simulink model "Saturation_Dynamic_verif"  (Simulink 7.2)
settings: Solver=ode45  StartTime=0.0  StopTime=10.0  RelTol=1e-3
libraries: simulink x1
settings Model: Creator=Romain  LastModifiedBy=Romain
settings OptimizationCC: ExpressionDepthLimit=128
settings DebuggingCC: SolverPrmCheckMsg=none  FcnCallInpInsideContextMsg=Enable All  StateNameClashWarn=none  StrictBusMsg=ErrorLevel1
settings CodeAppCC: CustomSymbolStrType=$N$R$M_T
settings GRTTargetCC: TargetFunctionLibrary=C89/C90 (ANSI)

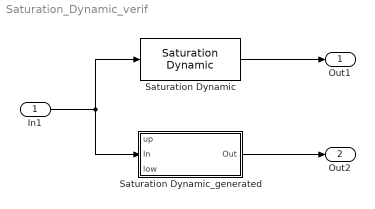
== system Saturation_Dynamic_verif ==
  In1 : Inport  OutDataTypeStr=double  DataType=double
  Saturation Dynamic : simulink/Discontinuities/Saturation Dynamic  OutMin=[]  OutMax=[]  OutDataTypeStr=Inherit: Same as second input  OutDataType=fixdt(1, 16)  OutScaling=2^-10  DoSatur=off
  Saturation Dynamic_generated : Subsystem  TreatAsAtomicUnit=on
  Out1 : Outport
  Out2 : Outport  Port=2
  wires:
  In1/1 -> Saturation Dynamic_generated/2(In), Saturation Dynamic/2
  Saturation Dynamic/1 -> Out1/1
  Saturation Dynamic_generated/1(Out) -> Out2/1

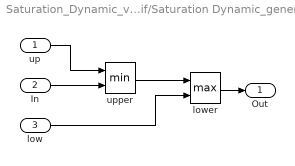
== system Saturation_Dynamic_verif/Saturation Dynamic_generated ==
  up : Inport
  In : Inport  Port=2
  low : Inport  Port=3
  lower : MinMax  Function=max  Inputs=2
  upper : MinMax  Inputs=2
  Out : Outport
  wires:
  up/1 -> upper/1
  upper/1 -> lower/1
  low/1 -> lower/2
  In/1 -> upper/2
  lower/1 -> Out/1
